simulink subsystem "MyModel"  (R2023a)
settings: Solver=VariableStepAuto  StartTime=0.0  StopTime=10.0  RelTol=1e-3
settings Model: Creator=KozlovM  LastModifiedBy=Алексей

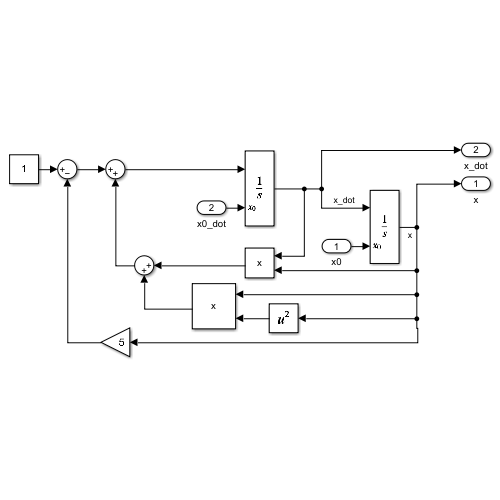
[thumbnail: Simulink's stored preview of the top-level diagram]
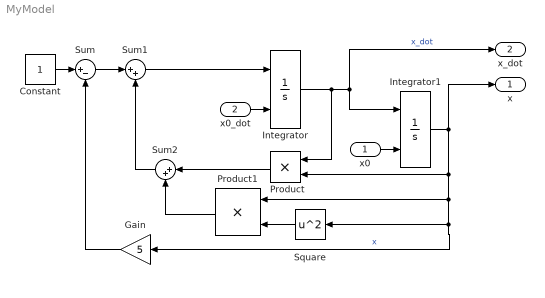
== system MyModel ==
  x0 : Inport
  x0_dot : Inport  Port=2
  Constant : Constant
  Gain : Gain  Gain=5
  Integrator : Integrator  InitialConditionSource=external
  Integrator1 : Integrator  InitialConditionSource=external
  Product : Product
  Product1 : Product
  Square : Math  Operator=square
  Sum : Sum  Inputs=|+-
  Sum1 : Sum  Inputs=|++
  Sum2 : Sum  Inputs=|++
  x : Outport
  x_dot : Outport  Port=2
  wires:
  Integrator1/1 -> x/1, Product1/1, Gain/1, Square/1, Product/2  "x"
  Integrator/1 -> Product/1, Integrator1/1, x_dot/1  "x_dot"
  x0_dot/1 -> Integrator/2
  x0/1 -> Integrator1/2
  Constant/1 -> Sum/1
  Gain/1 -> Sum/2
  Sum/1 -> Sum1/1
  Sum2/1 -> Sum1/2
  Sum1/1 -> Integrator/1
  Square/1 -> Product1/2
  Product/1 -> Sum2/1
  Product1/1 -> Sum2/2
